simulink model "model_bf_poi"  (Simulink 7.0)
settings: Solver=ode45  StartTime=0.0  StopTime=10.0  RelTol=1e-3
libraries: cstblocks x2
settings Model: Creator=fromion  LastModifiedBy=vfromion  ExtModeTrigMode=oneshot  ExtModeArmWhenConnect=off  ExtModeAutoUpdateStatusClock=off
settings DataIOCC: LimitDataPoints=off
settings OptimizationCC: BlockReduction=off  BooleanDataType=off
settings DebuggingCC: SaveWithParameterizedLinksMsg=none  SignalResolutionControl=TryResolveAllWithWarning  SolverPrmCheckMsg=none  MultiTaskDSMMsg=warning  MultiTaskCondExecSysMsg=none  StrictBusMsg=None
settings HardwareCC: TargetUnknown=on
settings RTWCC: IncludeERTFirstTime=on
settings GRTTargetCC: ModelReferenceCompliant=off  CompOptLevelCompliant=off  MatFileLogging=off

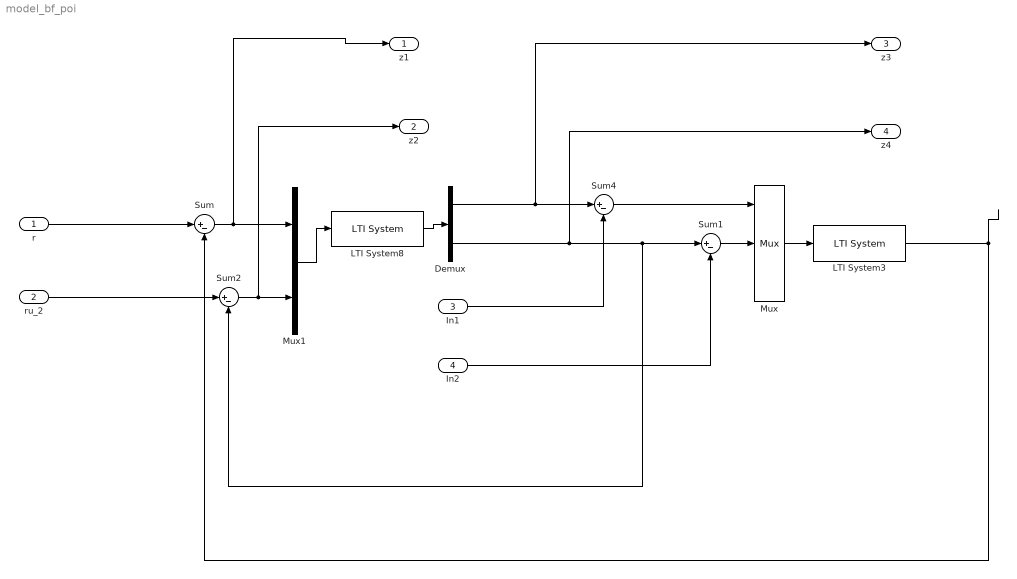
== system model_bf_poi ==
  r : Inport
  ru_2 : Inport  Port=2
  In1 : Inport  Port=3
  In2 : Inport  Port=4
  Demux : Demux  Outputs=2
  LTI System3 : cstblocks/LTI System  SystemSampleTime=-1  sys=sys_synt_ss  IC=0
  LTI System8 : cstblocks/LTI System  SystemSampleTime=-1  sys=K_hinf_ss  IC=0
  Mux : Mux  Inputs=3
  Mux1 : Mux  Inputs=2
  Sum{,1..2,4} (4 alike) : Sum  Inputs=|+-  SaturateOnIntegerOverflow=on  InputSameDT=on
  z1 : Outport
  z2 : Outport  Port=2
  z3 : Outport  Port=3
  z4 : Outport  Port=4
  wires:
  Sum/1 -> Mux1/1, z1/1
  In1/1 -> Sum4/2
  r/1 -> Sum/1
  LTI System3/1 -> Sum/2
  Sum4/1 -> Mux/1
  Demux/2 -> Sum1/1, Sum2/2, z4/1
  Sum1/1 -> Mux/2
  In2/1 -> Sum1/2
  ru_2/1 -> Sum2/1
  Sum2/1 -> Mux1/2, z2/1
  Mux/1 -> LTI System3/1
  Demux/1 -> Sum4/1, z3/1
  Mux1/1 -> LTI System8/1
  LTI System8/1 -> Demux/1
